simulink model "TP02"  (R2023a)
settings: Solver=ode1  StartTime=0.0  StopTime=100  FixedStep=5  RelTol=1e-3
undefined symbols (not defined in the file): g, K, l, ue, x0, xe
settings Model: Creator=pmt1554  LastModifiedBy=pmt1554

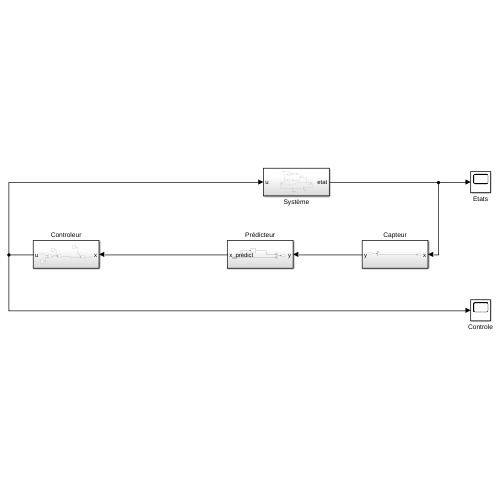
[thumbnail: Simulink's stored preview of the top-level diagram]
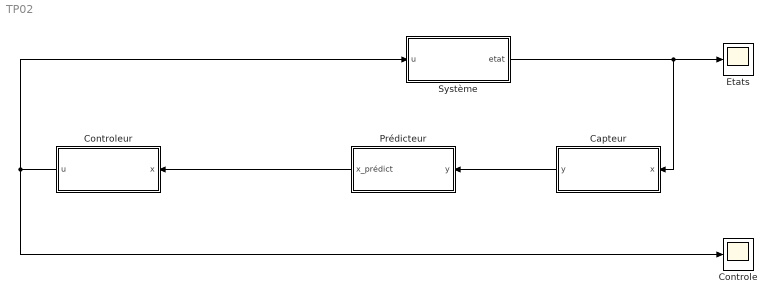
== system TP02 ==
  Capteur : Subsystem
  Controle : Scope
  Controleur : Subsystem
  Etats : Scope
  Prédicteur : Subsystem
  Système : Subsystem
  wires:
  Système/1(etat) -> Capteur/1(x), Etats/1
  Controleur/1(u) -> Controle/1, Système/1(u)
  Capteur/1(y) -> Prédicteur/1(y)
  Prédicteur/1(x_prédict) -> Controleur/1(x)

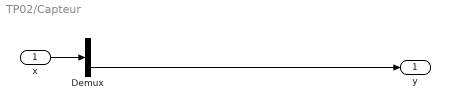
== system TP02/Capteur ==
  x : Inport
  Demux : Demux  Outputs=2
  y : Outport
  wires:
  x/1 -> Demux/1
  Demux/2 -> y/1

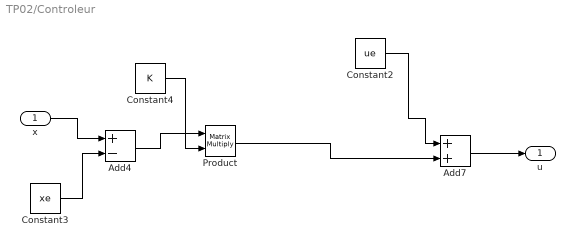
== system TP02/Controleur ==
  x : Inport
  Add4 : Sum  Inputs=+-
  Add7 : Sum
  Constant2 : Constant  Value=ue
  Constant3 : Constant  Value=xe
  Constant4 : Constant  Value=K
  Product : Product  Multiplication=Matrix(*)
  u : Outport
  wires:
  Product/1 -> Add7/2
  Constant2/1 -> Add7/1
  Add7/1 -> u/1
  x/1 -> Add4/1
  Constant3/1 -> Add4/2
  Constant4/1 -> Product/2
  Add4/1 -> Product/1

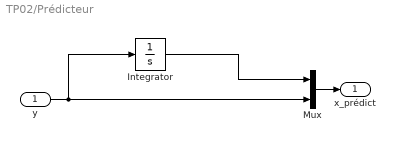
== system TP02/Prédicteur ==
  y : Inport
  Integrator : Integrator  InitialCondition=x0(1)
  Mux : Mux  Inputs=2
  x_prédict : Outport
  wires:
  Mux/1 -> x_prédict/1
  y/1 -> Integrator/1, Mux/2
  Integrator/1 -> Mux/1

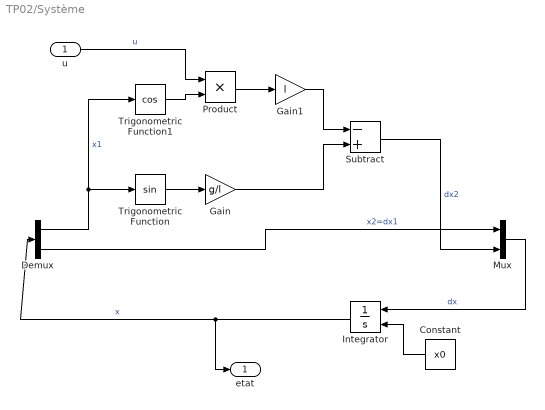
== system TP02/Système ==
  u : Inport
  Constant : Constant  Value=x0
  Demux : Demux  Outputs=2
  Gain : Gain  Gain=g/l
  Gain1 : Gain  Gain=l
  Integrator : Integrator  InitialConditionSource=external
  Mux : Mux  Inputs=2
  Product : Product
  Subtract : Sum  Inputs=-+
  Trigonometric Function : Trigonometry
  Trigonometric Function1 : Trigonometry  Operator=cos
  etat : Outport
  wires:
  Demux/2 -> Mux/1  "x2=dx1"
  Demux/1 -> Trigonometric Function1/1, Trigonometric Function/1  "x1"
  Trigonometric Function/1 -> Gain/1
  Mux/1 -> Integrator/1  "dx"
  Integrator/1 -> etat/1, Demux/1  "x"
  u/1 -> Product/1  "u"
  Trigonometric Function1/1 -> Product/2
  Product/1 -> Gain1/1
  Gain/1 -> Subtract/2
  Gain1/1 -> Subtract/1
  Subtract/1 -> Mux/2  "dx2"
  Constant/1 -> Integrator/2
